simulink library "AntiRollBar_None"  (R2022a)
settings: Solver=VariableStepAuto  StartTime=0.0  StopTime=10.0  RelTol=1e-3
libraries: sm_lib x3
Description:
  | Component of Simscape Vehicle Templates Library
  | 
  | Copyright 2018-2024 The MathWorks, Inc.
settings Model: Creator=smiller  LastModifiedBy=smiller
settings SolverCC: AlgebraicLoopSolver=TrustRegion
settings DataIOCC: ReturnWorkspaceOutputs=off
settings DebuggingCC: UnconnectedInputMsg=warning  UnconnectedOutputMsg=warning  UnconnectedLineMsg=warning  SFMachineParentedDataDiag=warning  ArithmeticOperatorsInVariantConditions=warning
settings SFSimCC: CustomCodeUndefinedFunction=UseInterfaceOnly
settings RTWCC: DLArmComputeVersion=19.05

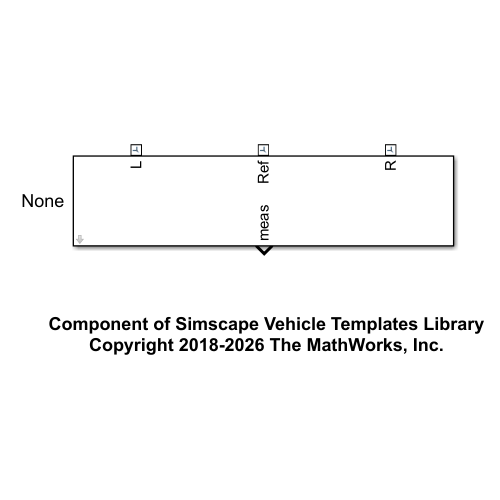
[thumbnail: Simulink's stored preview of the top-level diagram]
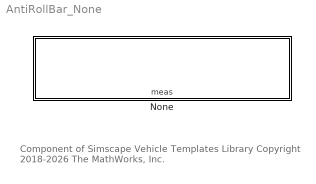
== system AntiRollBar_None ==
  note: Component of Simscape Vehicle Templates Library
      | Copyright 2018-2026 The MathWorks, Inc.
  " None" : Subsystem  VariantControl=None  mask(Anti-Roll Bar Placeholder){}
      mask help: Empty subsystem, used as a variant that omits an anti-roll bar.

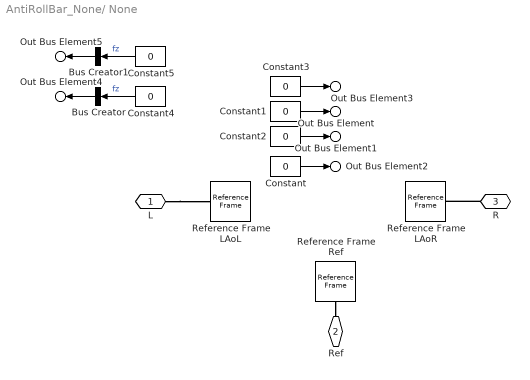
== system AntiRollBar_None/ None ==
  Bus Creator : BusCreator  Inputs=1
  Bus Creator1 : BusCreator  Inputs=1
  Constant{,1..5} (6 alike) : Constant  Value=0
  Reference Frame LAoL : sm_lib/Frames and Transforms/Reference Frame
  Reference Frame LAoR : sm_lib/Frames and Transforms/Reference Frame
  Reference Frame Ref : sm_lib/Frames and Transforms/Reference Frame
  L : PMIOPort  Side=Left
  Ref : PMIOPort  Port=2  Side=Left
  R : PMIOPort  Port=3  Side=Left
  Out Bus Element : Outport  VectorParamsAs1DForOutWhenUnconnected=off  PortName=meas  Element=zLA
  Out Bus Element1 : Outport  VectorParamsAs1DForOutWhenUnconnected=off  PortName=meas  Element=zRA
  Out Bus Element2 : Outport  VectorParamsAs1DForOutWhenUnconnected=off  PortName=meas  Element=fARB
  Out Bus Element3 : Outport  VectorParamsAs1DForOutWhenUnconnected=off  PortName=meas  Element=q
  Out Bus Element4 : Outport  VectorParamsAs1DForOutWhenUnconnected=off  PortName=meas  Element=MntL
  Out Bus Element5 : Outport  VectorParamsAs1DForOutWhenUnconnected=off  PortName=meas  Element=MntR
  wires:
  Constant/1 -> Out Bus Element2/1
  Constant1/1 -> Out Bus Element/1
  Constant2/1 -> Out Bus Element1/1
  Constant3/1 -> Out Bus Element3/1
  Bus Creator/1 -> Out Bus Element4/1
  Constant4/1 -> Bus Creator/1  "fz"
  Bus Creator1/1 -> Out Bus Element5/1
  Constant5/1 -> Bus Creator1/1  "fz"
  connections:
  Reference Frame Ref/RConn1 -- Ref/RConn1
  L/RConn1 -- Reference Frame LAoL/RConn1
  R/RConn1 -- Reference Frame LAoR/RConn1
